simulink model "FCElectricPlant"  (R2025b)
settings: Solver=VariableStepAuto  StartTime=0.0  StopTime=2474  RelTol=1e-3
model workspace (MAT data in the model file):
  Bat : object (value not decoded)
  BattDCDC : object (value not decoded)
  Brk : object (value not decoded)
  Cond : object (value not decoded)
  Cpl : object (value not decoded)
  DH2 = 74
  DH2O = 25
  DO2 = 18
  DRVctrl : object (value not decoded)
  Diff : object (value not decoded)
  Driveshaft : inertia (value not decoded)
  Duct : object (value not decoded)
  ElecThermal : object (value not decoded)
  FCDCDC : object (value not decoded)
  FCctrl : object (value not decoded)
  FTP72 : object (value not decoded)
  FTP75 : object (value not decoded)
  FinArea = 2
  FinDensity = 4
  H2_D = 74
  H2_R = 4124.48151676
  H2_T = [-56.55 -50 -40 -30 -20 -10 -5 -4 -3 -2 -1 0 ... (52 elements, 1x52)]
  H2_h = [2783.66044046 2873.94181646 3012.62601981 3152.22537302 3292.62486344 3433.7213836 3504.50184296 3518.67512521 3532.85394544 3547.03822323 3561.22787913 3575.42283463 ... (52 elements, 1x52)]
  H2_k = [142.834673487 146.602208511 152.236222043 157.732550942 163.09765294 168.338595937 170.914793442 171.426608923 171.937300227 172.446874689 172.955339635 173.462702375 ... (52 elements, 1x52)]
  H2_mu = [7.13280985169 7.28192581803 7.50683010986 7.72860158312 7.94743907375 8.16352107178 8.27057966039 8.29191522386 8.31322574339 8.33451136221 8.35577222214 8.37700846366 ... (52 elements, 1x52)]
  HWFET : object (value not decoded)
  Mot : object (value not decoded)
  N2_R = 296.802103844
  N2_T = [-56.55 -50 -40 -30 -20 -10 -5 -4 -3 -2 -1 0 ... (52 elements, 1x52)]
  N2_h = [224.312019476 231.141016529 241.564116975 251.984329606 262.402210767 272.818266127 278.025759131 279.06722248 280.10867517 281.150117667 282.191550441 283.232973957 ... (52 elements, 1x52)]
  N2_k = [19.6296532607 20.1533289725 20.9436243616 21.7231523445 22.4923063139 23.2514823267 23.6274403303 23.7023472872 23.7771601873 23.8518793809 23.9265052168 24.0010380424 ... (52 elements, 1x52)]
  N2_mu = [13.7948920665 14.1367187352 14.6513506072 15.1575394446 15.6556177861 16.1459023391 16.3882166949 16.4364580271 16.4846261831 16.532721447 16.5807441017 16.6286944287 ... (52 elements, 1x52)]
  NFin = 7680
  O2_D = 18
  O2_R = 259.836612623
  O2_T = [-56.55 -50 -40 -30 -20 -10 -5 -4 -3 -2 -1 0 ... (52 elements, 1x52)]
  O2_h = [196.314045635 202.302438243 211.445560194 220.590899229 229.740231593 238.895348953 243.475641264 244.39194743 245.308340402 246.224821996 247.14139403 248.05805832 ... (52 elements, 1x52)]
  O2_k = [19.6661951881 20.2224765128 21.0645207725 21.898029696 22.7232456338 23.5404090718 23.9460452976 24.0269406553 24.1077592592 24.1885013406 24.2691671302 24.349756858 ... (52 elements, 1x52)]
  O2_mu = [15.7665575307 16.1727626079 16.7849249434 17.3877315055 17.9815180942 18.5666055809 18.8559834763 18.9136105725 18.9711555252 19.0286186248 19.0860001607 19.1433004205 ... (52 elements, 1x52)]
  PTctrl : object (value not decoded)
  Pipe : object (value not decoded)
  Pump : object (value not decoded)
  RH2 = 4124.48291466
  RH2O = 461.523115726
  RH_a = 0.6
  RH_c = 0.6
  RN2 = 296.802204439
  RO2 = 259.836700689
  RelayVariant = 1
  ScenarioIndex = 5
  Sig : Simulink.Signal (value not decoded)
  SimEndTime = 2474
  T_cell = 80
  T_eff_bp = [0 20 40 60 80 100 120 140 160 180 200 220 ... (15 elements, 1x15)]
  T_env = 20
  T_ext = 30
  T_init = 303.15
  Tank : object (value not decoded)
  Tire : object (value not decoded)
  Tvec = [-50 -40 -30 -20 -10 0 10 20 30 40 50 60 ... (41 elements, 1x41)]
  US06 : object (value not decoded)
  UrbanCycle1 : object (value not decoded)
  UrbanCycle2 : object (value not decoded)
  UrbanCycle3 : object (value not decoded)
  UrbanCycle4 : object (value not decoded)
  UrbanCycle5 : object (value not decoded)
  Vehicle : object (value not decoded)
  WOT : object (value not decoded)
  anode_tube_D = 0.01
  cathode_tube_D = 0.05
  comp_mdot_corr_TLU = [0 0 0 0 0 0.2 0.15 0.1 0.05 0 0.4 0.3 ... (15 elements, 5x3)]
  comp_p_ratio_TLU = [1; 1.25; 1.5; 1.75; 2]
  comp_rpm_TLU = [0 1800 3600]
  coolant_num_layers = 20
  coolant_num_passes = 12
  coolant_tube_D = 0.05
  coolant_w_channels = 1
  drive_cycle_power = [0 0 0 0 0 0 0 0 0 0 0 0 ... (1050 elements, 1050x1)]
  drive_cycle_time = [0 3.15544362088e-30 0.0046730644306 0.0046730644306 0.0229169980413 0.0229169980413 0.0411609316521 0.0594048652628 0.0958927324843 0.168868466927 0.308339923682 0.308339923682 ... (1050 elements, 1050x1)]
  efficiency_table = [85 85 85 85 85 85 85 85 85 85 85 85 ... (180 elements, 12x15)]
  env_RH = 0.5
  env_T = 20
  env_p = 0.101325
  env_yO2 = 0.21
  f_fc_auxpower = [551.873653203 546.0853282 528.48462663 513.173595038 503.302975177 502.753456089 515.021163214 542.265022773 584.751680012 640.816461254 707.312051903 780.384247238 ... (869 elements, 79x11)]
  f_fc_currcmd_bpt = [0.209765 5.20060185897 10.1914387179 15.1822755769 20.1731124359 25.1639492949 30.1547861538 35.1456230128 40.1364598718 45.1272967308 50.1181335897 55.1089704487 ... (79 elements, 1x79)]
  f_fc_h2flow = [8.71593619412e-08 2.11208831613e-05 4.21802637945e-05 6.3315607286e-05 8.44733435522e-05 0.000105614873893 0.000126714989157 0.000147760022647 0.000168745833381 0.000189675717181 0.000210558338983 0.000231405772833 ... (869 elements, 79x11)]
  f_fc_heatflow = [-113.508553924 315.682858012 683.83093304 1077.33211881 1492.74924564 1928.28255982 2383.1090309 2856.86201514 3349.28475785 3860.05320307 4388.73420272 4934.82889994 ... (869 elements, 79x11)]
  f_fc_tmpcmd_bpt = [50 55 60 65 70 75 80 85 90 95 100]
  f_fc_voltage = [454.992615106 449.926167951 444.44198715 439.413829244 434.829610174 430.668984057 426.90491616 423.505302786 420.434569606 417.655187333 415.129053553 412.818701247 ... (869 elements, 79x11)]
  hH2 = [2873941.81645 3012626.01981 3152225.37301 3292624.86344 3433721.38359 3575422.83463 3717647.2553 3860321.98734 4003382.88163 4146773.54613 4290444.63593 4434353.18483 ... (41 elements, 1x41)]
  hH2O = [2407979.18389 2426599.35505 2445219.52621 2463839.69737 2482459.86853 2501080.03969 2520041.36444 2538661.5356 2557304.93352 2575974.09714 2594671.5511 2613399.77792 ... (41 elements, 1x41)]
  hN2 = [231141.016491 241564.116943 251984.329578 262402.210743 272818.266107 283232.973942 293646.803464 304060.22922 314473.742203 324887.858166 335303.123505 345720.119022 ... (41 elements, 1x41)]
  hO2 = [202302.438244 211445.560195 220590.89923 229740.231594 238895.348953 248058.05832 257230.174606 266413.508634 275609.852766 284820.965752 294048.557919 303294.277514 ... (41 elements, 1x41)]
  hvH2O = [2837864.0802 2838666.81899 2838713.54467 2838009.25742 2836579.406 2834477.18894 2477187.06302 2453519.25942 2429811.22988 2405977.28679 2381947.12654 2357654.5203 ... (41 elements, 1x41)]
  kH2 = [0.14660211438 0.15223611697 0.157732436203 0.163097529696 0.168338465237 0.173462565161 0.178477161614 0.183389433463 0.188206302164 0.192934369439 0.197579884152 0.202148729169 ... (41 elements, 1x41)]
  kH2O = [0.0133993325489 0.0140727292017 0.0147461258545 0.0154195225073 0.0160929191601 0.0167663158129 0.017416450238 0.0180898468908 0.0187835182831 0.019496836926 0.0202291830642 0.0209799564979 ... (41 elements, 1x41)]
  kN2 = [0.0201533289599 0.0209436243479 0.0217231523299 0.0224923062983 0.0232514823103 0.0240010380251 0.0247413260421 0.0254726839711 0.026195434744 0.0269098870397 0.0276163357829 0.028315062687 ... (41 elements, 1x41)]
  kO2 = [0.0202224764979 0.0210645207571 0.0218980296803 0.0227232456176 0.0235404090551 0.0243497568408 0.0251515209302 0.0259459275017 0.0267331962527 0.0275135401488 0.0282871691008 0.0290542796888 ... (41 elements, 1x41)]
  muH2 = [7.28192631884e-06 7.50683062629e-06 7.72860211493e-06 7.94743962074e-06 8.16352163375e-06 8.37700904042e-06 8.58804741514e-06 8.79676894741e-06 9.00329407235e-06 9.20773285791e-06 9.41018619135e-06 9.61074679906e-06 ... (41 elements, 1x41)]
  muH2O = [7.40754821278e-06 7.71570492949e-06 8.0238616462e-06 8.33201836291e-06 8.64017507962e-06 8.94833179633e-06 9.24231634895e-06 9.55047306566e-06 9.87031914628e-06 1.02003383346e-05 1.05392900589e-05 1.08861429187e-05 ... (41 elements, 1x41)]
  muN2 = [1.41367187228e-05 1.46513505944e-05 1.51575394313e-05 1.56556177724e-05 1.6145902325e-05 1.66286944141e-05 1.71042805521e-05 1.75729330776e-05 1.80349108304e-05 1.84904598363e-05 1.89398139868e-05 1.9383195703e-05 ... (41 elements, 1x41)]
  muO2 = [1.6172762594e-05 1.67849249289e-05 1.73877314906e-05 1.79815180788e-05 1.8566605565e-05 1.9143300404e-05 1.97118951916e-05 2.02726692488e-05 2.08258892185e-05 2.13718096611e-05 2.19106736419e-05 2.24427133044e-05 ... (41 elements, 1x41)]
  pH2O = [0.0039376926592 0.0128411282011 0.0380050105363 0.103238678713 0.259872929049 0.611151401419 1.22819893069 2.33931818334 4.24697083683 7.38493807375 12.3519458375 19.9464343078 ... (41 elements, 1x41)]
  p_a = 0.101325
  p_c = 0.101325
  p_sat = 0.0474144740302
  p_sat_c = 0.0474144740302
  p_sat_e = 0.00233931818334
  radiator_H = 0.5
  radiator_L = 1
  radiator_N_fins = 12000
  radiator_N_tubes = 25
  radiator_W = 0.025
  radiator_air_area_fins = 11.5625
  radiator_air_area_primary = 1.223125
  radiator_cp = 910
  radiator_eta_fin = 0.7
  radiator_fin_spacing = 0.002
  radiator_gap_H = 0.0192708333333
  radiator_rho = 2700
  radiator_t_wall = 0.0001
  radiator_tube_H = 0.0015
  radiator_tube_Leq = 2.5
  stack_D_gdl = 0.07
  stack_alpha = 0.6
  stack_area = 280
  stack_iL = 1.4
  stack_io = 0.0001
  stack_mea_cp = 870
  stack_mea_rho = 1800
  stack_membrane_MW = 1.1
  stack_membrane_rho = 2000
  stack_num_cells = 400
  stack_num_channels = 8
  stack_t_gdl = 250
  stack_t_membrane = 125
  stack_w_channels = 1
  tank_V = 120
  tank_p = 70
  tank_yH2 = 0.9997
  y_H2O_a = 0.280766685597
  y_H2O_c = 0.0138523652603
  y_H2_a = 0.719233314403
  y_N2_a = 0
  y_N2_c = 0.77614763474
  y_O2_c = 0.21
symbols that are objects in the model workspace (value not decoded): Bat, ElecThermal, Mot
libraries: fl_lib x91, nesl_utility x43, autolibpowerinfoutils x9, SimscapeFluids_lib x5, ee_lib x3, slpidlib x2, batteryecm_lib x1, simulink_extras x1, simulink x1
(part 3 of 4)

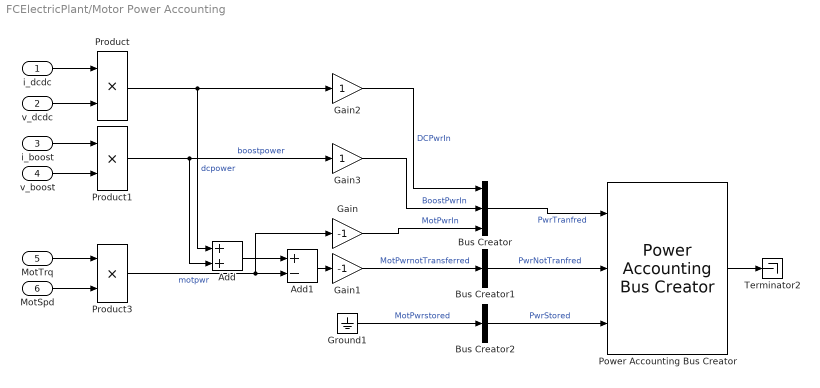
== system FCElectricPlant/Motor Power Accounting ==
  i_dcdc : Inport
  v_dcdc : Inport  Port=2
  i_boost : Inport  Port=3
  v_boost : Inport  Port=4
  MotTrq : Inport  Port=5
  MotSpd : Inport  Port=6
  Add : Sum
  Add1 : Sum  Inputs=+-
  Bus Creator : BusCreator  Inputs=3
  Bus Creator1 : BusCreator  Inputs=1
  Bus Creator2 : BusCreator  Inputs=1
  Gain : Gain  Gain=-1
  Gain1 : Gain  Gain=-1
  Gain2 : Gain
  Gain3 : Gain
  Ground1 : Ground
  Power Accounting Bus Creator : autolibpowerinfoutils/Power Accounting Bus Creator  AssctBlkSelPopup=Parent  RefBlkName='autolibsharedcoupling/Torsional Compliance'  PwrTrnsfrdCheckBox=on  PwrNotTrnsfrdCheckBox=on  PwrStoredCheckBox=on  aMode=aMode
  Product : Product
  Product1 : Product
  Product3 : Product
  Terminator2 : Terminator
  wires:
  Gain3/1 -> Bus Creator/2  "BoostPwrIn"
  Gain2/1 -> Bus Creator/1  "DCPwrIn"
  Product/1 -> Add/1, Gain2/1  "dcpower"
  Product1/1 -> Add/2, Gain3/1  "boostpower"
  v_boost/1 -> Product1/2
  i_boost/1 -> Product1/1
  v_dcdc/1 -> Product/2
  i_dcdc/1 -> Product/1
  Bus Creator/1 -> Power Accounting Bus Creator/1  "PwrTranfred"
  Gain/1 -> Bus Creator/3  "MotPwrIn"
  Power Accounting Bus Creator/1 -> Terminator2/1
  Ground1/1 -> Bus Creator2/1  "MotPwrstored"
  Add1/1 -> Gain1/1
  MotTrq/1 -> Product3/1
  MotSpd/1 -> Product3/2
  Bus Creator1/1 -> Power Accounting Bus Creator/2  "PwrNotTranfred"
  Bus Creator2/1 -> Power Accounting Bus Creator/3  "PwrStored"
  Product3/1 -> Gain/1, Add1/2  "motpwr"
  Add/1 -> Add1/1
  Gain1/1 -> Bus Creator1/1  "MotPwrnotTransferred"

== system FCElectricPlant/Subsystem1 ==
  AmbTemp : Inport
  Controlled Temperature Source1 : fl_lib/Thermal/Thermal Sources/Controlled Temperature Source
  Simulink-PS Converter2 : nesl_utility/Simulink-PS Converter  PhysicalDomain=network_engine_domain  SubClassName=ps_input  LeftPortType=input  RightPortType=output  PseudoPeriodic=off  Frequencies=[]  NoiseDistribution=none  NoiseParameters=[]  Unit=K  AffineConversion=on  FilteringAndDerivatives=provide  SimscapeFilterOrder=1  InputFilterTimeConstant=0.001  UdotUserProvided=0
  Thermal Reference3 : fl_lib/Thermal/Thermal Elements/Thermal Reference
  B : PMIOPort  Side=Right
  wires:
  AmbTemp/1 -> Simulink-PS Converter2/1
  connections:
  Simulink-PS Converter2/RConn1 -- Controlled Temperature Source1/RConn1
  Thermal Reference3/LConn1 -- Controlled Temperature Source1/RConn2
  Controlled Temperature Source1/LConn1 -- B/RConn1

== system FCElectricPlant/Battery System/Power Acc ==
  P_Acc : Inport
  VBatt : Inport  Port=2
  Controlled Current Source : fl_lib/Electrical/Electrical Sources/Controlled Current Source
  Divide : Product  Inputs=*/
  Saturation : Saturate  UpperLimit=inf  LowerLimit=min(Bat.noLoadV, [], 'all')  ZeroCross=off
  Simulink-PS Converter : nesl_utility/Simulink-PS Converter  PhysicalDomain=network_engine_domain  SubClassName=ps_input  LeftPortType=input  RightPortType=output  PseudoPeriodic=off  Frequencies=[]  NoiseDistribution=none  NoiseParameters=[]  Unit=A  AffineConversion=off  FilteringAndDerivatives=filter  SimscapeFilterOrder=1  InputFilterTimeConstant=0.001  UdotUserProvided=0
  + : PMIOPort  Side=Left
  - : PMIOPort  Port=2  Side=Right
  wires:
  Saturation/1 -> Divide/2
  Divide/1 -> Simulink-PS Converter/1
  P_Acc/1 -> Divide/1
  VBatt/1 -> Saturation/1
  connections:
  Simulink-PS Converter/RConn1 -- Controlled Current Source/RConn1
  +/RConn1 -- Controlled Current Source/RConn2
  -/RConn1 -- Controlled Current Source/LConn1

== system FCElectricPlant/Battery System/Sensor VI ==
  Bus Creator : BusCreator  Inputs=2
  Current Sensor : fl_lib/Electrical/Electrical Sensors/Current Sensor
  PS-Simulink Converter2 : nesl_utility/PS-Simulink Converter  PhysicalDomain=network_engine_domain  SubClassName=ps_output  LeftPortType=input  RightPortType=output  PseudoPeriodic=off  Frequencies=[]  VectorFormat=1-D array  Unit=1  AffineConversion=off
  PS-Simulink Converter4 : nesl_utility/PS-Simulink Converter  PhysicalDomain=network_engine_domain  SubClassName=ps_output  LeftPortType=input  RightPortType=output  PseudoPeriodic=off  Frequencies=[]  VectorFormat=1-D array  Unit=1  AffineConversion=off
  Transfer Fcn5 : TransferFcn  Denominator=[0.001 1]
  Voltage Sensor2 : fl_lib/Electrical/Electrical Sensors/Voltage Sensor
  + : PMIOPort  Side=Left
  - : PMIOPort  Port=2  Side=Right
  G : PMIOPort  Port=3  Side=Right
  vi : Outport
  wires:
  Bus Creator/1 -> vi/1
  PS-Simulink Converter4/1 -> Transfer Fcn5/1
  PS-Simulink Converter2/1 -> Bus Creator/2  "BattCurr"
  Transfer Fcn5/1 -> Bus Creator/1  "BattV"
  connections:
  Current Sensor/RConn1 -- PS-Simulink Converter2/LConn1
  Voltage Sensor2/RConn2 -- G/RConn1
  Current Sensor/RConn2 -- -/RConn1
  PS-Simulink Converter4/LConn1 -- Voltage Sensor2/RConn1
  Voltage Sensor2/LConn1 -- Current Sensor/LConn1 -- +/RConn1

== system FCElectricPlant/Battery System/Sensor VI1 ==
  Current Sensor : fl_lib/Electrical/Electrical Sensors/Current Sensor
  PS-Simulink Converter4 : nesl_utility/PS-Simulink Converter  PhysicalDomain=network_engine_domain  SubClassName=ps_output  LeftPortType=input  RightPortType=output  PseudoPeriodic=off  Frequencies=[]  VectorFormat=1-D array  Unit=1  AffineConversion=off
  Transfer Fcn (with initial outputs) : simulink_extras/Additional Linear/Transfer Fcn (with initial outputs)  N=[1]  D="[0.001  1]"  Y0=FCDCDC.Vout  U0=FCDCDC.Vout
  Voltage Sensor2 : fl_lib/Electrical/Electrical Sensors/Voltage Sensor
  + : PMIOPort  Side=Left
  I : PMIOPort  Port=2  Side=Right
  - : PMIOPort  Port=3  Side=Right
  G : PMIOPort  Port=4  Side=Right
  HVDC : Outport
  v_dcdc : Outport  Port=2
  wires:
  PS-Simulink Converter4/1 -> v_dcdc/1, Transfer Fcn (with initial outputs)/1
  Transfer Fcn (with initial outputs)/1 -> HVDC/1  "HVDC"
  connections:
  +/RConn1 -- Current Sensor/LConn1 -- Voltage Sensor2/LConn1
  PS-Simulink Converter4/LConn1 -- Voltage Sensor2/RConn1
  Current Sensor/RConn2 -- -/RConn1
  Voltage Sensor2/RConn2 -- G/RConn1
  I/RConn1 -- Current Sensor/RConn1

== system FCElectricPlant/Battery System/Thermal ==
  v_dcdc : Inport
  Controlled Heat Flow Rate Source : fl_lib/Thermal/Thermal Sources/Controlled Heat Flow Rate Source
  PS Gain : fl_lib/Physical Signals/Functions/PS Gain  gain=0.001 Ohm
  PS Math Function : fl_lib/Physical Signals/Functions/PS Math Function  fcn_choice=foundation.enum.math_function.square  v=1
  PS-Simulink Converter : nesl_utility/PS-Simulink Converter  PhysicalDomain=network_engine_domain  SubClassName=ps_output  LeftPortType=input  RightPortType=output  PseudoPeriodic=off  Frequencies=[]  VectorFormat=inherit  Unit=inherit  AffineConversion=off
  Product : Product
  Thermal Mass : fl_lib/Thermal/Thermal Elements/Thermal Mass  mass_type=foundation.enum.constant_variable.constant  mass=15 kg  sp_heat=447 J/kg/K  mass_min=1e-6 kg  num_ports=foundation.enum.numPorts2.one  m_specify=off  m_priority=High  m=1 kg  m_nominal_specify=off  m_nominal_value=1  m_nominal_unit=kg  T_specify=off  T_priority=High  T=300 K  T_nominal_specify=off  T_nominal_value=1  T_nominal_unit=K  Q_specify=off  Q_priority=None  Q=0 W  Q_nominal_specify=off  Q_nominal_value=1  Q_nominal_unit=W
  Thermal Resistance : fl_lib/Thermal/Thermal Elements/Thermal Resistance  resistance=0.1 K/W  T_specify=off  T_priority=None  T=0 K  T_nominal_specify=off  T_nominal_value=1  T_nominal_unit=K  Q_specify=off  Q_priority=None  Q=0 W  Q_nominal_specify=off  Q_nominal_value=1  Q_nominal_unit=W
  Thermal Reference3 : fl_lib/Thermal/Thermal Elements/Thermal Reference
  H : PMIOPort  Side=Right
  i : PMIOPort  Port=2  Side=Left
  pwr_dcdc : Outport
  i_dcdc : Outport  Port=2
  wires:
  PS-Simulink Converter/1 -> i_dcdc/1, Product/1  "i_dcdc"
  Product/1 -> pwr_dcdc/1
  v_dcdc/1 -> Product/2  "v_dcdc"
  connections:
  PS Gain/RConn1 -- Controlled Heat Flow Rate Source/RConn1
  i/RConn1 -- PS-Simulink Converter/LConn1 -- PS Math Function/LConn1
  H/RConn1 -- Thermal Resistance/RConn1
  Thermal Reference3/LConn1 -- Controlled Heat Flow Rate Source/RConn2
  PS Gain/LConn1 -- PS Math Function/RConn1
  Controlled Heat Flow Rate Source/LConn1 -- Thermal Mass/LConn1 -- Thermal Resistance/LConn1

== system FCElectricPlant/Cooling System Power Analysis/Heat Exchanger Power Accounting ==
  P3 : Inport
  Phe : Inport  Port=2
  P4 : Inport  Port=3
  Add : Sum  Inputs=++-
  Bus Creator : BusCreator  Inputs=2
  Bus Creator1 : BusCreator  Inputs=2
  Gain1 : Gain
  Gain2 : Gain  Gain=-1
  Gain3 : Gain  Gain=-1
  Power Accounting Bus Creator : autolibpowerinfoutils/Power Accounting Bus Creator  AssctBlkSelPopup=Parent  RefBlkName='autolibsharedcoupling/Torsional Compliance'  PwrTrnsfrdCheckBox=on  PwrNotTrnsfrdCheckBox=on  PwrStoredCheckBox=off  aMode=aMode
  Terminator2 : Terminator
  wires:
  Bus Creator/1 -> Power Accounting Bus Creator/1  "PwrTranfred"
  P3/1 -> Bus Creator/1, Add/2  "InternalEnergyIn"
  Power Accounting Bus Creator/1 -> Terminator2/1
  Phe/1 -> Add/1, Gain1/1
  Bus Creator1/1 -> Power Accounting Bus Creator/2  "PwrNotTranfred"
  P4/1 -> Gain2/1, Add/3
  Gain2/1 -> Bus Creator/2  "InternalEnergyOut"
  Add/1 -> Gain3/1  "Pdiff"
  Gain3/1 -> Bus Creator1/2  "PowerNotTransferred1"
  Gain1/1 -> Bus Creator1/1  "HeatDissipated"

== system FCElectricPlant/Cooling System Power Analysis/Pipe Converter Power Accounting ==
  P1 : Inport
  Pfc : Inport  Port=2
  P2 : Inport  Port=3
  Add : Sum  Inputs=++-
  Bus Creator : BusCreator  Inputs=2
  Bus Creator1 : BusCreator  Inputs=2
  Gain1 : Gain
  Gain2 : Gain  Gain=-1
  Gain3 : Gain  Gain=-1
  Power Accounting Bus Creator : autolibpowerinfoutils/Power Accounting Bus Creator  AssctBlkSelPopup=Parent  RefBlkName='autolibsharedcoupling/Torsional Compliance'  PwrTrnsfrdCheckBox=on  PwrNotTrnsfrdCheckBox=on  PwrStoredCheckBox=off  aMode=aMode
  Terminator2 : Terminator
  wires:
  Gain3/1 -> Bus Creator1/2  "PowerNotTransferred1"
  Add/1 -> Gain3/1  "Pdiff"
  Gain2/1 -> Bus Creator/2  "InternalEnergyOut"
  P2/1 -> Add/3, Gain2/1
  Bus Creator1/1 -> Power Accounting Bus Creator/2  "PwrNotTranfred"
  Pfc/1 -> Gain1/1, Add/1  "HeatDissipated"
  Power Accounting Bus Creator/1 -> Terminator2/1
  P1/1 -> Bus Creator/1, Add/2  "InternalEnergyIn"
  Bus Creator/1 -> Power Accounting Bus Creator/1  "PwrTranfred"
  Gain1/1 -> Bus Creator1/1  "HeatDissipated"

== system FCElectricPlant/Cooling System Power Analysis/Pipe Motor Power Accounting ==
  P2 : Inport
  Ptcm : Inport  Port=2
  P3 : Inport  Port=3
  Add : Sum  Inputs=++-
  Bus Creator : BusCreator  Inputs=2
  Bus Creator1 : BusCreator  Inputs=2
  Gain1 : Gain
  Gain2 : Gain  Gain=-1
  Gain3 : Gain  Gain=-1
  Power Accounting Bus Creator : autolibpowerinfoutils/Power Accounting Bus Creator  AssctBlkSelPopup=Parent  RefBlkName='autolibsharedcoupling/Torsional Compliance'  PwrTrnsfrdCheckBox=on  PwrNotTrnsfrdCheckBox=on  PwrStoredCheckBox=off  aMode=aMode
  Terminator2 : Terminator
  wires:
  Gain3/1 -> Bus Creator1/2  "PowerNotTransferred1"
  Add/1 -> Gain3/1  "P diff"
  Gain2/1 -> Bus Creator/2  "InternalEnergyOut"
  P3/1 -> Gain2/1, Add/3
  Bus Creator1/1 -> Power Accounting Bus Creator/2  "PwrNotTrnsfrd"
  Ptcm/1 -> Add/2, Gain1/1  "HeatDissipated"
  Power Accounting Bus Creator/1 -> Terminator2/1
  P2/1 -> Bus Creator/1, Add/1  "InternalEnergyIn"
  Bus Creator/1 -> Power Accounting Bus Creator/1  "PwrTrnsfrd"
  Gain1/1 -> Bus Creator1/1  "HeatDissipated"

== system FCElectricPlant/Cooling System Power Analysis/Tank Power Accounting ==
  P4 : Inport
  Pconv : Inport  Port=2
  P1 : Inport  Port=3
  Add : Sum  Inputs=++-
  Bus Creator : BusCreator  Inputs=2
  Bus Creator1 : BusCreator  Inputs=2
  Gain1 : Gain
  Gain2 : Gain  Gain=-1
  Gain3 : Gain  Gain=-1
  Power Accounting Bus Creator : autolibpowerinfoutils/Power Accounting Bus Creator  AssctBlkSelPopup=Parent  RefBlkName='autolibsharedcoupling/Torsional Compliance'  PwrTrnsfrdCheckBox=on  PwrNotTrnsfrdCheckBox=on  PwrStoredCheckBox=off  aMode=aMode
  Terminator2 : Terminator
  wires:
  Gain3/1 -> Bus Creator1/2  "PowerNotTransferred1"
  Add/1 -> Gain3/1  "Pdiff"
  Gain2/1 -> Bus Creator/2  "InternalEnergyOut"
  P1/1 -> Add/3, Gain2/1
  Bus Creator1/1 -> Power Accounting Bus Creator/2  "PwrNotTrnsfrd"
  Pconv/1 -> Add/1, Gain1/1  "HeatDissipated"
  Power Accounting Bus Creator/1 -> Terminator2/1
  P4/1 -> Bus Creator/1, Add/2  "InternalEnergyIn"
  Bus Creator/1 -> Power Accounting Bus Creator/1  "PwrTrnsfrd"
  Gain1/1 -> Bus Creator1/1  "HeatDissipated"

== system FCElectricPlant/Electrical Cooling System/Heat flow sensor ==
  Heat Flow Rate Sensor2 : fl_lib/Thermal/Thermal Sensors/Heat Flow Rate Sensor
  PS-Simulink Converter2 : nesl_utility/PS-Simulink Converter  PhysicalDomain=network_engine_domain  SubClassName=ps_output  LeftPortType=input  RightPortType=output  PseudoPeriodic=off  Frequencies=[]  VectorFormat=inherit  Unit=inherit  AffineConversion=off
  Temperature Sensor : fl_lib/Thermal/Thermal Sensors/Temperature Sensor  temperature_measure=foundation.enum.MeasurementReference.difference
  Thermal Reference : fl_lib/Thermal/Thermal Elements/Thermal Reference
  B : PMIOPort  Side=Right
  A : PMIOPort  Port=2  Side=Left
  tag scope: Phe=global
  wires:
  PS-Simulink Converter2/1 -> [Phe]  "Phe"
  connections:
  Heat Flow Rate Sensor2/RConn1 -- PS-Simulink Converter2/LConn1
  Heat Flow Rate Sensor2/RConn2 -- Temperature Sensor/LConn1 -- B/RConn1
  A/RConn1 -- Heat Flow Rate Sensor2/LConn1
  Temperature Sensor/RConn1 -- Thermal Reference/LConn1

== system FCElectricPlant/Electrical Cooling System/Heat flow sensor1 ==
  Goto1 : Goto  Commented=on  GotoTag=Tconv  TagVisibility=global
  Heat Flow Rate Sensor2 : fl_lib/Thermal/Thermal Sensors/Heat Flow Rate Sensor
  PS-Simulink Converter1 : nesl_utility/PS-Simulink Converter  Commented=on  PhysicalDomain=network_engine_domain  SubClassName=ps_output  LeftPortType=input  RightPortType=output  PseudoPeriodic=off  Frequencies=[]  VectorFormat=1-D array  Unit=K  AffineConversion=off
  PS-Simulink Converter2 : nesl_utility/PS-Simulink Converter  PhysicalDomain=network_engine_domain  SubClassName=ps_output  LeftPortType=input  RightPortType=output  PseudoPeriodic=off  Frequencies=[]  VectorFormat=inherit  Unit=inherit  AffineConversion=off
  Temperature Sensor : fl_lib/Thermal/Thermal Sensors/Temperature Sensor  temperature_measure=foundation.enum.MeasurementReference.difference
  Thermal Reference : fl_lib/Thermal/Thermal Elements/Thermal Reference
  B : PMIOPort  Side=Right
  A : PMIOPort  Port=2  Side=Left
  tag scope: Pconv=global
  wires:
  PS-Simulink Converter1/1 -> Goto1/1
  PS-Simulink Converter2/1 -> [Pconv]  "Pconv"
  connections:
  Temperature Sensor/RConn1 -- Thermal Reference/LConn1
  Temperature Sensor/RConn2 -- PS-Simulink Converter1/LConn1
  A/RConn1 -- Heat Flow Rate Sensor2/LConn1
  Temperature Sensor/LConn1 -- B/RConn1 -- Heat Flow Rate Sensor2/RConn2
  Heat Flow Rate Sensor2/RConn1 -- PS-Simulink Converter2/LConn1

== system FCElectricPlant/Electrical Cooling System/Pump Control ==
  TAmb : Inport
  TMotor : Inport  Port=2
  Add : Sum  Inputs=|-+
  PID Controller : slpidlib/PID Controller  Controller=PI  Form=Parallel  TimeDomain=Continuous-time  UseExternalTs=off  SampleTime=-1  IntegratorMethod=Forward Euler  FilterMethod=Forward Euler  ControllerParametersSource=internal  P=ElecThermal.ctrl.Kp  I=ElecThermal.ctrl.Ki  UseKiTs=off  D=0  UseExternalDerivativeSource=off  N=100  UseFilter=on  TunerSelectOption=Transfer Function Based (PID Tuner App)  ZeroCross=off  InitialConditionSource=internal  InitialConditionForIntegrator=0  InitialConditionForFilter=0  DifferentiatorICPrevScaledInput=0  ExternalReset=none  TrackingMode=off  Kt=1  LimitOutput=on  SatLimitsSource=internal  UpperSaturationLimit=0.1  LowerSaturationLimit=0  LinearizeAsGain=on  AntiWindupMode=clamping  Kb=1  LimitIntegrator=off  UpperIntegratorSaturationLimit=inf  LowerIntegratorSaturationLimit=-inf  POutMin=[]  POutMax=[]  IOutMin=[]  IOutMax=[]  DOutMin=[]  DOutMax=[]  NOutMin=[]  NOutMax=[]  SumOutMin=[]  SumOutMax=[]  SaturationOutMin=[]  SaturationOutMax=[]  PParamMin=[]  PParamMax=[]  IParamMin=[]  IParamMax=[]  DParamMin=[]  DParamMax=[]  NParamMin=[]  NParamMax=[]  KbParamMin=[]  KbParamMax=[]  KtParamMin=[]  KtParamMax=[]  KbOutMin=[]  KbOutMax=[]  KtOutMin=[]  KtOutMax=[]  IntegratorOutMin=[]  IntegratorOutMax=[]  FilterOutMin=[]  FilterOutMax=[]  SumI1OutMin=[]  SumI1OutMax=[]  SumI2OutMin=[]  SumI2OutMax=[]  SumI3OutMin=[]  SumI3OutMax=[]  SumI4OutMin=[]  SumI4OutMax=[]  SumDOutMin=[]  SumDOutMax=[]  DifferentiatorOutMin=[]  DifferentiatorOutMax=[]  FilterDiffOutCoefMin=[]  FilterDiffOutCoefMax=[]  ReciprocalOutMin=[]  ReciprocalOutMax=[]  SumDenOutMin=[]  SumDenOutMax=[]  SumNumOutMin=[]  SumNumOutMax=[]  DivideOutMin=[]  DivideOutMax=[]  UdiffTsProdOutMin=[]  UdiffTsProdOutMax=[]  NTsProdOutMin=[]  NTsProdOutMax=[]  UintegralTsProdOutMin=[]  UintegralTsProdOutMax=[]  UngainTsProdOutMin=[]  UngainTsProdOutMax=[]  ClampingZeroOutDataTypeStr=Inherit: Inherit via back propagation  ClampingZeroOutMin=[]  ClampingZeroOutMax=[]  FilterDenConstantOutDataTypeStr=Inherit: Inherit via back propagation  FilterDenConstantOutMin=[]  FilterDenConstantOutMax=[]  PCopyOutDataTypeStr=Inherit: Inherit via back propagation  PCopyOutMin=[]  PCopyOutMax=[]  NCopyOutDataTypeStr=Inherit: Inherit via back propagation  NCopyOutMin=[]  NCopyOutMax=[]  IntegratorContinuousStateAttributes=''  IntegratorStateMustResolveToSignalObject=off  IntegratorRTWStateStorageClass=Auto  FilterContinuousStateAttributes=''  FilterStateMustResolveToSignalObject=off  FilterRTWStateStorageClass=Auto  ParallelPVariant=InternalParameters  IdealPVariant=Disabled  IVariant=InternalParameters  DVariant=Disabled  IntegratorVariant=Continuous  SatVariant=Enabled  AWVariant=ContClampingParallel  PCopyVariant=Disabled  TRVariant=Disabled  FdbkBlocksVariant=Forward  IdealPFdbkVariant=Disabled  SatFdbkVariant=Disabled  DerivativeFilterVariant=Disabled  NVariant=Disabled  NCopyVariant=Disabled_SignalSpec  FilterICVariant=Disabled  IntegratorICVariant=InternalICs  ExternalResetVariant=Disabled  TRSumVariant=Passthrough  SumFdbkVariant=Disabled  SumVariant=Sum_PI  TsampFilterVariant=InternalTs  TsampNgainVariant=Passthrough  TsampIntegralVariant=Disabled_SignalSpec  ExternalSaturationOutDataTypeStr=Inherit: Same as second input  DerivativeSourceVariant=Disabled  PreIntVariant=InternalPreInt
  Sensor Dynamics : TransferFcn  Denominator=[0.1 1]
  Sensor Dynamics1 : TransferFcn  Denominator=[0.1 1]
  Pump_flw : Outport
  wires:
  TMotor/1 -> Sensor Dynamics/1
  TAmb/1 -> Sensor Dynamics1/1
  PID Controller/1 -> Pump_flw/1  "Pump_flw"
  Add/1 -> PID Controller/1
  Sensor Dynamics/1 -> Add/2
  Sensor Dynamics1/1 -> Add/1

== system FCElectricPlant/Electrical Cooling System/Sensing T Amb ==
  PS-Simulink Converter1 : nesl_utility/PS-Simulink Converter  PhysicalDomain=network_engine_domain  SubClassName=ps_output  LeftPortType=input  RightPortType=output  PseudoPeriodic=off  Frequencies=[]  VectorFormat=1-D array  Unit=K  AffineConversion=off
  Temperature Sensor : fl_lib/Thermal/Thermal Sensors/Temperature Sensor  temperature_measure=foundation.enum.MeasurementReference.difference
  Thermal Reference : fl_lib/Thermal/Thermal Elements/Thermal Reference
  A : PMIOPort  Side=Left
  T : Outport
  wires:
  PS-Simulink Converter1/1 -> T/1
  connections:
  Temperature Sensor/RConn1 -- Thermal Reference/LConn1
  Temperature Sensor/RConn2 -- PS-Simulink Converter1/LConn1
  Temperature Sensor/LConn1 -- A/RConn1

== system FCElectricPlant/Electrical Cooling System/Sensing T MotorR ==
  PS-Simulink Converter1 : nesl_utility/PS-Simulink Converter  PhysicalDomain=network_engine_domain  SubClassName=ps_output  LeftPortType=input  RightPortType=output  PseudoPeriodic=off  Frequencies=[]  VectorFormat=1-D array  Unit=K  AffineConversion=off
  Temperature Sensor : fl_lib/Thermal/Thermal Sensors/Temperature Sensor  temperature_measure=foundation.enum.MeasurementReference.difference
  Thermal Reference : fl_lib/Thermal/Thermal Elements/Thermal Reference
  A : PMIOPort  Side=Left
  T : Outport
  wires:
  PS-Simulink Converter1/1 -> T/1
  connections:
  Temperature Sensor/LConn1 -- A/RConn1
  Temperature Sensor/RConn2 -- PS-Simulink Converter1/LConn1
  Temperature Sensor/RConn1 -- Thermal Reference/LConn1

== system FCElectricPlant/Electrical Cooling System/Sensors ==
  Abs : Abs  ZeroCross=off  SaturateOnIntegerOverflow=off
  Average Efficiency : fl_lib/Physical Signals/Sources/PS Constant  constant=0.9
  PS Divide : fl_lib/Physical Signals/Functions/PS Divide
  PS Product : fl_lib/Physical Signals/Functions/PS Product
  PS-Simulink Converter : nesl_utility/PS-Simulink Converter  PhysicalDomain=network_engine_domain  SubClassName=ps_output  LeftPortType=input  RightPortType=output  PseudoPeriodic=off  Frequencies=[]  VectorFormat=1-D array  Unit=inherit  AffineConversion=off
  Pressure & Temperature Sensor (TL) : fl_lib/Thermal Liquid/Sensors/Pressure & Temperature Sensor (TL)  reference=foundation.enum.MeasurementReference.difference  pressure=true  pressure_spec=foundation.enum.PressureMeasementSpec.Absolute  temperature=true
      settings: InternalSimscapePortConfiguration="{\"Bottom\":[{\"id\":\"T\",\"label\":\"T\",\"type\":\"output\"}],\"Left\":[{\"id\":\"A\",\"label\":\"A\",\"type\":\"foundation.thermal_liquid.thermal_liquid\"}],\"Right\":[{\"id\":\"B\",\"label\":\"B\",\"type\":\"foundation.thermal_liquid.thermal_liquid\"},{\"id\":\"P\",\"label\":\"P\",\"type\":\"output\"}],\"Top\":[]}"
  Transfer Fcn3 : TransferFcn  Denominator=[0.001 1]
  Volumetric Flow Rate Sensor (TL) : fl_lib/Thermal Liquid/Sensors/Flow Rate Sensor (TL)  mass_flow_measure=false  volumetric_flow_measure=true  energy_flow_measure=false
      settings: InternalSimscapePortConfiguration="{\"Bottom\":[],\"Left\":[{\"id\":\"A\",\"label\":\"A\",\"type\":\"foundation.thermal_liquid.thermal_liquid\"}],\"Right\":[{\"id\":\"B\",\"label\":\"B\",\"type\":\"foundation.thermal_liquid.thermal_liquid\"},{\"id\":\"V\",\"label\":\"V\",\"type\":\"output\"}],\"Top\":[]}"
  B : PMIOPort  Side=Left
  A : PMIOPort  Port=2  Side=Right
  A_P : PMIOPort  Port=3  Side=Right
  Power : Outport
  wires:
  PS-Simulink Converter/1 -> Abs/1
  Abs/1 -> Transfer Fcn3/1
  Transfer Fcn3/1 -> Power/1
  connections:
  Pressure & Temperature Sensor (TL)/RConn1 -- Volumetric Flow Rate Sensor (TL)/RConn1 -- B/RConn1
  PS Product/LConn1 -- Pressure & Temperature Sensor (TL)/RConn2
  Volumetric Flow Rate Sensor (TL)/RConn2 -- PS Product/LConn2
  PS Divide/LConn1 -- PS Product/RConn1
  Average Efficiency/RConn1 -- PS Divide/LConn2
  PS-Simulink Converter/LConn1 -- PS Divide/RConn1
  A_P/RConn1 -- Pressure & Temperature Sensor (TL)/LConn1
  A/RConn1 -- Volumetric Flow Rate Sensor (TL)/LConn1

== system FCElectricPlant/Electrical Cooling System/Tank ==
  Absolute Reference (TL) : fl_lib/Thermal Liquid/Elements/Absolute Reference (TL)
  Cap (G) : fl_lib/Gas/Elements/Cap (G)  p_specify=off  p_priority=None  p=0.101325 MPa  p_nominal_specify=off  p_nominal_value=1  p_nominal_unit=MPa  T_specify=off  T_priority=None  T=293.15 K  T_nominal_specify=off  T_nominal_value=1  T_nominal_unit=K
  Convection HGas : fl_lib/Thermal/Thermal Elements/Convective Heat Transfer  thermal_type=foundation.enum.constant_variable.constant  area=1e-2 m^2  heat_tr_coeff=20 W/(m^2 * K)  min_heat_tr_coeff=1e-3 W/(K*m^2)  T_specify=off  T_priority=None  T=0 K  T_nominal_specify=off  T_nominal_value=1  T_nominal_unit=K  Q_specify=off  Q_priority=None  Q=0 W  Q_nominal_specify=off  Q_nominal_value=1  Q_nominal_unit=W
  Convection HLiq : fl_lib/Thermal/Thermal Elements/Convective Heat Transfer  thermal_type=foundation.enum.constant_variable.constant  area=1e-4 m^2  heat_tr_coeff=20 W/(m^2 * K)  min_heat_tr_coeff=1e-3 W/(K*m^2)  T_specify=off  T_priority=None  T=0 K  T_nominal_specify=off  T_nominal_value=1  T_nominal_unit=K  Q_specify=off  Q_priority=None  Q=0 W  Q_nominal_specify=off  Q_nominal_value=1  Q_nominal_unit=W
  Flow Resistance (G) : fl_lib/Gas/Elements/Flow Resistance (G)  delta_p_nominal=0.001 MPa  mdot_nominal=0.1 kg/s  rho_nominal=0 kg/m^3  area=ElecThermal.Tank.areaVectorA1B1(1) m^2  laminar_fraction=1e-3
      settings: InternalSimscapePortConfiguration="{\"Bottom\":[],\"Left\":[{\"id\":\"A\",\"label\":\"A\",\"type\":\"foundation.gas.gas\"}],\"Right\":[{\"id\":\"B\",\"label\":\"B\",\"type\":\"foundation.gas.gas\"}],\"Top\":[]}"
  PS-Simulink Converter1 : nesl_utility/PS-Simulink Converter  PhysicalDomain=network_engine_domain  SubClassName=ps_output  LeftPortType=input  RightPortType=output  PseudoPeriodic=off  Frequencies=[]  VectorFormat=1-D array  Unit=K  AffineConversion=off
  Reservoir (G) : fl_lib/Gas/Elements/Reservoir (G)  pressure_spec=foundation.enum.pressure_spec.atmospheric  reservoir_pressure=0.101325 MPa  reservoir_temperature=300 K  area_A=ElecThermal.Tank.areaVectorA1B1(1) m^2
  Sensor P T : fl_lib/Thermal Liquid/Sensors/Pressure & Temperature Sensor (TL)  reference=foundation.enum.MeasurementReference.difference  pressure=true  pressure_spec=foundation.enum.PressureMeasementSpec.Absolute  temperature=true
      settings: InternalSimscapePortConfiguration="{\"Bottom\":[{\"id\":\"T\",\"label\":\"T\",\"type\":\"output\"}],\"Left\":[{\"id\":\"A\",\"label\":\"A\",\"type\":\"foundation.thermal_liquid.thermal_liquid\"}],\"Right\":[{\"id\":\"B\",\"label\":\"B\",\"type\":\"foundation.thermal_liquid.thermal_liquid\"},{\"id\":\"P\",\"label\":\"P\",\"type\":\"output\"}],\"Top\":[]}"
  Tank : SimscapeFluids_lib/Thermal Liquid/Tanks & Accumulators/Tank (G-TL)  num_inlet=fluids.thermal_liquid.tanks_accumulators.enum.NumInlet.Two  volume_total=ElecThermal.Tank.volume m^3  volume_spec=1  tank_area=ElecThermal.Tank.area m^2  level_TLU=[0, 3, 5] m  volume_TLU=[0, 4, 6] m^3  inlet_areas_A1B1=ElecThermal.Tank.areaVectorA1B1 m^2  inlet_height_A2=0.1 m  inlet_area_A2=0.01 m^2  inlet_heights_A2B2=ElecThermal.Tank.heightVector m  inlet_areas_A2B2=ElecThermal.Tank.areaVectorA2B2 m^2  inlet_heights_A2B2C2=[.1, .1, .1] m  inlet_areas_A2B2C2=[.01, .01, .01] m^2  inlet_heights_A2B2C2D2=0.1 * ones(1, 4) m  inlet_areas_A2B2C2D2=0.01 * ones(1, 4) m^2  inlet_heights_A2B2C2D2E2=0.1 * ones(1, 5) m  inlet_areas_A2B2C2D2E2=0.01 * ones(1, 5) m^2  inlet_heights_A2B2C2D2E2F2=0.1 * ones(1, 6) m  inlet_areas_A2B2C2D2E2F2=0.01 * ones(1, 6) m^2  capacity_check=1  max_liquid_capacity=ElecThermal.Tank.volume m^3  g=9.81 m/s^2  level_specify=on  level_priority=High  level=0.1 m  level_nominal_specify=off  level_nominal_value=1  level_nominal_unit=m  volume_liquid_specify=off  volume_liquid_priority=None  volume_liquid=5 m^3  volume_liquid_nominal_specify=off  volume_liquid_nominal_value=1  volume_liquid_nominal_unit=m^3  mass_liquid_specify=off  mass_liquid_priority=None  mass_liquid=5e+3 kg  mass_liquid_nominal_specify=off  mass_liquid_nominal_value=1  mass_liquid_nominal_unit=kg  T_liquid_specify=on  T_liquid_priority=High  T_liquid=300 K  T_liquid_nominal_specify=off  T_liquid_nominal_value=1  T_liquid_nominal_unit=K  p_gas_specify=off  p_gas_priority=High  p_gas=0.101325 MPa  p_gas_nominal_specify=off  p_gas_nominal_value=1  p_gas_nominal_unit=MPa  T_gas_specify=on  T_gas_priority=High  T_gas=300 K  T_gas_nominal_specify=off  T_gas_nominal_value=1  T_gas_nominal_unit=K  rho_gas_specify=off  rho_gas_priority=None  rho_gas=1.2 kg/m^3  rho_gas_nominal_specify=off  rho_gas_nominal_value=1  rho_gas_nominal_unit=kg/m^3
      settings: InternalSimscapePortConfiguration="{\"Bottom\":[],\"Left\":[{\"id\":\"A1\",\"label\":\"A1\",\"type\":\"foundation.gas.gas\"},{\"id\":\"B1\",\"label\":\"B1\",\"type\":\"foundation.gas.gas\"},{\"id\":\"A2\",\"label\":\"A2\",\"type\":\"foundation.thermal_liquid.thermal_liquid\"},{\"id\":\"B2\",\"label\":\"B2\",\"type\":\"foundation.thermal_liquid.thermal_liquid\"}],\"Right\":[{\"id\":\"H1\",\"label\":\"H1\",\"type\":\"foundation.thermal.thermal\"},{\"id\":\"H2\",\"label\":\"H2\",\"type\":\"foundation.thermal.thermal\"}],\"Top\":[{\"id\":\"V_out\",\"label\":\"V\",\"type\":\"output\"},{\"id\":\"L_out\",\"label\":\"L\",\"type\":\"output\"}]}"
  Terminator2 : Terminator
  B : PMIOPort  Side=Left
  HGas : PMIOPort  Port=2  Side=Left
  A : PMIOPort  Port=3  Side=Right
  HLiq : PMIOPort  Port=4  Side=Left
  wires:
  PS-Simulink Converter1/1 -> Terminator2/1
  connections:
  Convection HLiq/RConn1 -- HLiq/RConn1
  PS-Simulink Converter1/LConn1 -- Sensor P T/RConn3
  Sensor P T/RConn1 -- Absolute Reference (TL)/LConn1
  B/RConn1 -- Sensor P T/LConn1 -- Tank/LConn4
  Cap (G)/LConn1 -- Tank/LConn2
  Convection HGas/RConn1 -- HGas/RConn1
  Reservoir (G)/LConn1 -- Flow Resistance (G)/LConn1
  Tank/LConn3 -- A/RConn1
  Flow Resistance (G)/RConn1 -- Tank/LConn1
  Tank/RConn2 -- Convection HLiq/LConn1
  Convection HGas/LConn1 -- Tank/RConn1

== system FCElectricPlant/Electrical Cooling System/Thermal Circuit Converter FC ==
  Conductive Heat Transfer : fl_lib/Thermal/Thermal Elements/Conductive Heat Transfer  thermal_type=foundation.enum.ConstantVariableTabulated.Constant  wall_geometry=foundation.enum.ConductionWallGeometry.Planar  area=0.01*pi*1 m^2  thickness=0.004 m  d_in=0.05 m  d_out=0.1 m  L=1 m  th_cond_min=10 W/(K*m)  th_cond="237;  %Al W/(m*K)"  th_cond_TLU=[413, 401, 392, 383, 371, 357, 342] W/(K*m)  temp_TLU=[200, 273, 400, 600, 800, 1000, 1200] K  T_specify=off  T_priority=None  T=0 K  T_nominal_specify=off  T_nominal_value=1  T_nominal_unit=K  Q_specify=off  Q_priority=None  Q=0 W  Q_nominal_specify=off  Q_nominal_value=1  Q_nominal_unit=W
  Heat Flow Rate Sensor : fl_lib/Thermal/Thermal Sensors/Heat Flow Rate Sensor
  PS-Simulink Converter4 : nesl_utility/PS-Simulink Converter  PhysicalDomain=network_engine_domain  SubClassName=ps_output  LeftPortType=input  RightPortType=output  PseudoPeriodic=off  Frequencies=[]  VectorFormat=inherit  Unit=inherit  AffineConversion=off
  Temperature Sensor : fl_lib/Thermal/Thermal Sensors/Temperature Sensor  temperature_measure=foundation.enum.MeasurementReference.difference
  Thermal Mass : fl_lib/Thermal/Thermal Elements/Thermal Mass  mass_type=foundation.enum.constant_variable.constant  mass=ElecThermal.TM1.mass kg  sp_heat=ElecThermal.TM1.sh J/kg/K  mass_min=1e-6 kg  num_ports=foundation.enum.numPorts2.one  m_specify=off  m_priority=High  m=1 kg  m_nominal_specify=off  m_nominal_value=1  m_nominal_unit=kg  T_specify=off  T_priority=High  T=300 K  T_nominal_specify=off  T_nominal_value=1  T_nominal_unit=K  Q_specify=off  Q_priority=High  Q=0 W  Q_nominal_specify=off  Q_nominal_value=1  Q_nominal_unit=W
  Thermal Reference : fl_lib/Thermal/Thermal Elements/Thermal Reference
  A : PMIOPort  Side=Left
  B : PMIOPort  Port=2  Side=Right
  tag scope: Pfc=global
  wires:
  PS-Simulink Converter4/1 -> [Pfc]  "Pfc"
  connections:
  Conductive Heat Transfer/LConn1 -- A/RConn1
  Conductive Heat Transfer/RConn1 -- Thermal Mass/LConn1 -- Temperature Sensor/LConn1 -- Heat Flow Rate Sensor/LConn1
  B/RConn1 -- Heat Flow Rate Sensor/RConn2
  PS-Simulink Converter4/LConn1 -- Heat Flow Rate Sensor/RConn1
  Temperature Sensor/RConn1 -- Thermal Reference/LConn1

== system FCElectricPlant/Electrical Cooling System/Thermal Circuit Motor ==
  Case-Ambient Insulated : fl_lib/Thermal/Thermal Elements/Perfect Insulator  T_specify=off  T_priority=None  T=0 K  T_nominal_specify=off  T_nominal_value=1  T_nominal_unit=K
  Heat Flow Rate Sensor : fl_lib/Thermal/Thermal Sensors/Heat Flow Rate Sensor
  Iron Stack-Case Conductance : fl_lib/Thermal/Thermal Elements/Conductive Heat Transfer  thermal_type=foundation.enum.ConstantVariableTabulated.Constant  wall_geometry=foundation.enum.ConductionWallGeometry.Planar  area=Mot.ironStack.area cm^2  thickness=Mot.ironStack.thick cm  d_in=0.05 m  d_out=0.1 m  L=1 m  th_cond_min=10 W/(K*m)  th_cond=Mot.ironStack.cond W/(m*K)  th_cond_TLU=[413, 401, 392, 383, 371, 357, 342] W/(K*m)  temp_TLU=[200, 273, 400, 600, 800, 1000, 1200] K  T_specify=off  T_priority=None  T=0 K  T_nominal_specify=off  T_nominal_value=1  T_nominal_unit=K  Q_specify=off  Q_priority=None  Q=0 W  Q_nominal_specify=off  Q_nominal_value=1  Q_nominal_unit=W
  Motor Case Thermal Mass : fl_lib/Thermal/Thermal Elements/Thermal Mass  mass_type=foundation.enum.constant_variable.constant  mass=Mot.ironStack.mass kg  sp_heat=Mot.ironStack.sh J/kg/K  mass_min=1e-6 kg  num_ports=foundation.enum.numPorts2.one  m_specify=off  m_priority=High  m=1 kg  m_nominal_specify=off  m_nominal_value=1  m_nominal_unit=kg  T_specify=off  T_priority=High  T=300 K  T_nominal_specify=off  T_nominal_value=1  T_nominal_unit=K  Q_specify=off  Q_priority=None  Q=0 W  Q_nominal_specify=off  Q_nominal_value=1  Q_nominal_unit=W
  PS-Simulink Converter4 : nesl_utility/PS-Simulink Converter  PhysicalDomain=network_engine_domain  SubClassName=ps_output  LeftPortType=input  RightPortType=output  PseudoPeriodic=off  Frequencies=[]  VectorFormat=inherit  Unit=inherit  AffineConversion=off
  Stator Iron Thermal Mass : fl_lib/Thermal/Thermal Elements/Thermal Mass  mass_type=foundation.enum.constant_variable.constant  mass=Mot.windingIron.mass kg  sp_heat=Mot.windingIron.sh J/kg/K  mass_min=1e-6 kg  num_ports=foundation.enum.numPorts2.one  m_specify=off  m_priority=High  m=1 kg  m_nominal_specify=off  m_nominal_value=1  m_nominal_unit=kg  T_specify=off  T_priority=High  T=300 K  T_nominal_specify=off  T_nominal_value=1  T_nominal_unit=K  Q_specify=off  Q_priority=None  Q=0 W  Q_nominal_specify=off  Q_nominal_value=1  Q_nominal_unit=W
  Winding Conductance : fl_lib/Thermal/Thermal Elements/Conductive Heat Transfer  thermal_type=foundation.enum.ConstantVariableTabulated.Constant  wall_geometry=foundation.enum.ConductionWallGeometry.Planar  area=Mot.winding.area cm^2  thickness=Mot.winding.thick cm  d_in=0.05 m  d_out=0.1 m  L=1 m  th_cond_min=10 W/(K*m)  th_cond=Mot.winding.cond W/(m*K)  th_cond_TLU=[413, 401, 392, 383, 371, 357, 342] W/(K*m)  temp_TLU=[200, 273, 400, 600, 800, 1000, 1200] K  T_specify=off  T_priority=None  T=0 K  T_nominal_specify=off  T_nominal_value=1  T_nominal_unit=K  Q_specify=off  Q_priority=None  Q=0 W  Q_nominal_specify=off  Q_nominal_value=1  Q_nominal_unit=W
  Winding Thermal Mass : fl_lib/Thermal/Thermal Elements/Thermal Mass  mass_type=foundation.enum.constant_variable.constant  mass=Mot.winding.mass kg  sp_heat=Mot.winding.sh J/kg/K  mass_min=1e-6 kg  num_ports=foundation.enum.numPorts2.one  m_specify=off  m_priority=High  m=1 kg  m_nominal_specify=off  m_nominal_value=1  m_nominal_unit=kg  T_specify=off  T_priority=High  T=300 K  T_nominal_specify=off  T_nominal_value=1  T_nominal_unit=K  Q_specify=off  Q_priority=None  Q=0 W  Q_nominal_specify=off  Q_nominal_value=1  Q_nominal_unit=W
  Winding-Iron Conductance : fl_lib/Thermal/Thermal Elements/Conductive Heat Transfer  thermal_type=foundation.enum.ConstantVariableTabulated.Constant  wall_geometry=foundation.enum.ConductionWallGeometry.Planar  area=Mot.windingIron.area cm^2  thickness=Mot.windingIron.thick cm  d_in=0.05 m  d_out=0.1 m  L=1 m  th_cond_min=10 W/(K*m)  th_cond=Mot.windingIron.cond W/(m*K)  th_cond_TLU=[413, 401, 392, 383, 371, 357, 342] W/(K*m)  temp_TLU=[200, 273, 400, 600, 800, 1000, 1200] K  T_specify=off  T_priority=None  T=0 K  T_nominal_specify=off  T_nominal_value=1  T_nominal_unit=K  Q_specify=off  Q_priority=None  Q=0 W  Q_nominal_specify=off  Q_nominal_value=1  Q_nominal_unit=W
  A : PMIOPort  Side=Left
  B : PMIOPort  Port=2  Side=Right
  tag scope: Ptcm=global
  wires:
  PS-Simulink Converter4/1 -> [Ptcm]  "Ptcm"
  connections:
  Winding Conductance/LConn1 -- Winding-Iron Conductance/RConn1 -- Winding Thermal Mass/LConn1
  Motor Case Thermal Mass/LConn1 -- Iron Stack-Case Conductance/RConn1 -- Case-Ambient Insulated/LConn1
  Stator Iron Thermal Mass/LConn1 -- Winding-Iron Conductance/LConn1 -- Heat Flow Rate Sensor/LConn1 -- Iron Stack-Case Conductance/LConn1
  Winding Conductance/RConn1 -- A/RConn1
  PS-Simulink Converter4/LConn1 -- Heat Flow Rate Sensor/RConn1
  Heat Flow Rate Sensor/RConn2 -- B/RConn1

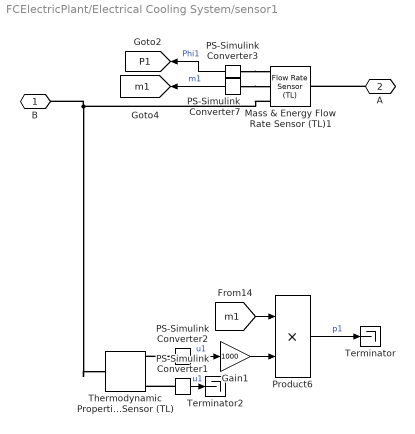
== system FCElectricPlant/Electrical Cooling System/sensor1 ==
  Gain1 : Gain  Gain=1000
  Mass & Energy Flow Rate Sensor (TL)1 : fl_lib/Thermal Liquid/Sensors/Flow Rate Sensor (TL)  mass_flow_measure=true  volumetric_flow_measure=false  energy_flow_measure=true
      settings: InternalSimscapePortConfiguration="{\"Bottom\":[{\"id\":\"PHI\",\"label\":\"φ\",\"type\":\"output\"}],\"Left\":[{\"id\":\"A\",\"label\":\"A\",\"type\":\"foundation.thermal_liquid.thermal_liquid\"}],\"Right\":[{\"id\":\"B\",\"label\":\"B\",\"type\":\"foundation.thermal_liquid.thermal_liquid\"},{\"id\":\"M\",\"label\":\"M\",\"type\":\"output\"}],\"Top\":[]}"
  PS-Simulink Converter{1..3,7} (4 alike) : nesl_utility/PS-Simulink Converter  PhysicalDomain=network_engine_domain  SubClassName=ps_output  LeftPortType=input  RightPortType=output  PseudoPeriodic=off  Frequencies=[]  VectorFormat=inherit  Unit=inherit  AffineConversion=off
  Product6 : Product
  Terminator : Terminator
  Terminator2 : Terminator
  Thermodynamic Properties Sensor (TL) : fl_lib/Thermal Liquid/Sensors/Thermodynamic Properties Sensor (TL)  internal_energy=true  density=true  specific_heat=true
      settings: InternalSimscapePortConfiguration="{\"Bottom\":[],\"Left\":[{\"id\":\"A\",\"label\":\"A\",\"type\":\"foundation.thermal_liquid.thermal_liquid\"}],\"Right\":[{\"id\":\"U\",\"label\":\"u\",\"type\":\"output\"},{\"id\":\"RHO\",\"label\":\"ρ\",\"type\":\"output\"},{\"id\":\"CP\",\"label\":\"cp\",\"type\":\"output\"}],\"Top\":[]}"
  B : PMIOPort  Side=Left
  A : PMIOPort  Port=2  Side=Right
  tag scope: P1=global, m1=global
  wires:
  PS-Simulink Converter7/1 -> [m1]  "m1"
  Product6/1 -> Terminator/1  "p1"
  Gain1/1 -> Product6/2
  PS-Simulink Converter2/1 -> Gain1/1  "u1"
  [m1] -> Product6/1
  PS-Simulink Converter1/1 -> Terminator2/1  "u1"
  PS-Simulink Converter3/1 -> [P1]  "Phi1"
  connections:
  A/RConn1 -- Mass & Energy Flow Rate Sensor (TL)1/LConn1
  PS-Simulink Converter7/LConn1 -- Mass & Energy Flow Rate Sensor (TL)1/RConn2
  Mass & Energy Flow Rate Sensor (TL)1/RConn1 -- Thermodynamic Properties Sensor (TL)/LConn1 -- B/RConn1
  PS-Simulink Converter2/LConn1 -- Thermodynamic Properties Sensor (TL)/RConn1
  PS-Simulink Converter1/LConn1 -- Thermodynamic Properties Sensor (TL)/RConn3
  PS-Simulink Converter3/LConn1 -- Mass & Energy Flow Rate Sensor (TL)1/RConn3
